simulink model "initializejoystick_model"  (Simulink 6.4)
settings: Solver=ode4  StartTime=0.0  StopTime=0.02*100  FixedStep=0.02  RelTol=1e-3
libraries: aerosimlib x1, RT x1
Description:
  | This model is be used with InitializeJoystick.m in order to obtain appropriate zero offsets and gains for the joystick interface.
settings Model: Creator=Christopher Lum  LastModifiedBy=root
settings DataIOCC: SignalLoggingName=sigsOut
settings DebuggingCC: SolverPrmCheckMsg=none  StrictBusMsg=None
settings HardwareCC: TargetUnknown=on

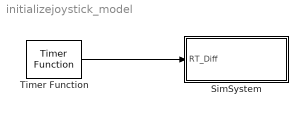
== system initializejoystick_model ==
  SimSystem : Subsystem
  Timer Function : RT/Timer Function  Priority=264547656  step=20  priority=HIGH  ThPriority=NORMAL
  wires:
  Timer Function/1 -> SimSystem/1(RT_Diff)

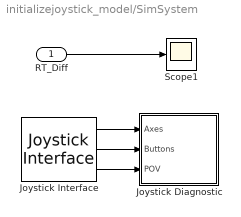
== system initializejoystick_model/SimSystem ==
  RT_Diff : Inport
  Joystick Diagnostic : Subsystem
  Joystick Interface : aerosimlib/Pilot Interface/Joystick Interface  SystemSampleTime=-1  joyid=1  tsamp=0.02
  Scope1 : Scope
      settings: YMin=0  YMax=4500
  wires:
  RT_Diff/1 -> Scope1/1
  Joystick Interface/1 -> Joystick Diagnostic/1(Axes)
  Joystick Interface/2 -> Joystick Diagnostic/2(Buttons)
  Joystick Interface/3 -> Joystick Diagnostic/3(POV)

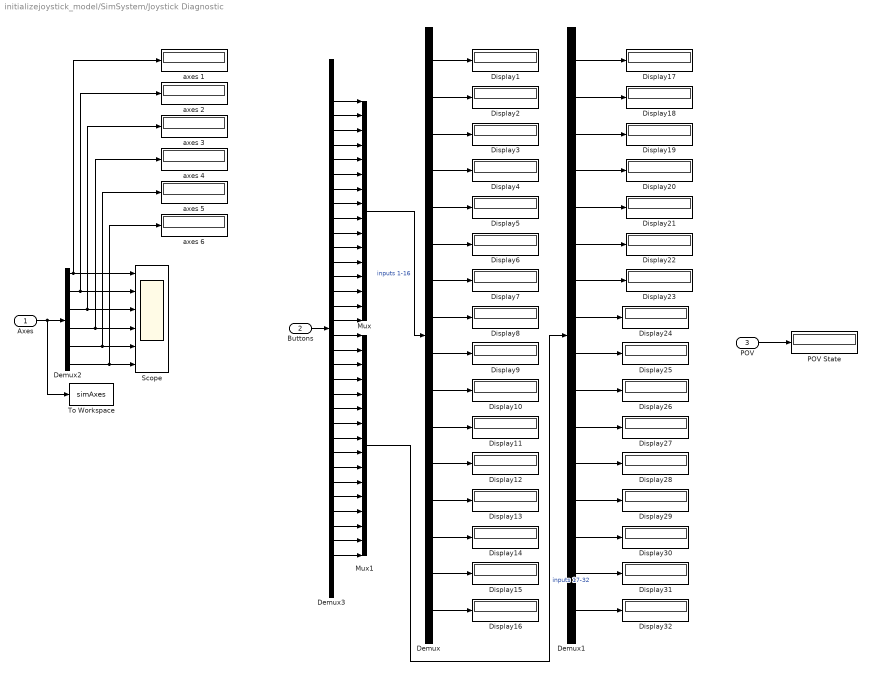
== system initializejoystick_model/SimSystem/Joystick Diagnostic ==
  Axes : Inport
  Buttons : Inport  Port=2
  POV : Inport  Port=3
  Demux : Demux  Outputs=16
  Demux1 : Demux  Outputs=16
  Demux2 : Demux  Outputs=6
  Demux3 : Demux  Outputs=32
  Display{1..32} (32 alike) : Display
  Mux : Mux  Inputs=16
  Mux1 : Mux  Inputs=16
  POV State : Display
  Scope : Scope  NumInputPorts=6
      settings: YMin=30885.5~30885.5~62258.3~-1~-1~-1  YMax=34136.6~34136.6~68811.8~1~1~1
  To Workspace : ToWorkspace  VariableName=simAxes  SampleTime=-1  SaveFormat=Structure With Time
  axes {1..6} (6 alike) : Display
  wires:
  Buttons/1 -> Demux3/1
  Demux3/1 -> Mux/1
  Demux3/2 -> Mux/2
  Demux3/3 -> Mux/3
  Demux3/4 -> Mux/4
  Demux3/5 -> Mux/5
  Demux3/6 -> Mux/6
  Demux3/7 -> Mux/7
  Demux3/8 -> Mux/8
  Demux3/9 -> Mux/9
  Demux3/10 -> Mux/10
  Demux3/11 -> Mux/11
  Demux3/12 -> Mux/12
  Demux3/13 -> Mux/13
  Demux3/14 -> Mux/14
  Demux3/15 -> Mux/15
  Demux3/16 -> Mux/16
  Mux/1 -> Demux/1  "inputs 1-16"
  Demux3/17 -> Mux1/1
  Demux3/18 -> Mux1/2
  Demux3/19 -> Mux1/3
  Demux3/20 -> Mux1/4
  Demux3/21 -> Mux1/5
  Demux3/22 -> Mux1/6
  Demux3/23 -> Mux1/7
  Demux3/24 -> Mux1/8
  Demux3/25 -> Mux1/9
  Demux3/26 -> Mux1/10
  Demux3/27 -> Mux1/11
  Demux3/28 -> Mux1/12
  Demux3/29 -> Mux1/13
  Demux3/30 -> Mux1/14
  Demux3/31 -> Mux1/15
  Demux3/32 -> Mux1/16
  Mux1/1 -> Demux1/1  "inputs 17-32"
  Demux/1 -> Display1/1
  Demux/2 -> Display2/1
  Demux/3 -> Display3/1
  Demux/4 -> Display4/1
  Demux/5 -> Display5/1
  Demux/6 -> Display6/1
  Demux/7 -> Display7/1
  Demux/8 -> Display8/1
  Demux/9 -> Display9/1
  Demux/10 -> Display10/1
  Demux/11 -> Display11/1
  Demux/12 -> Display12/1
  Demux/13 -> Display13/1
  Demux/14 -> Display14/1
  Demux/15 -> Display15/1
  Demux/16 -> Display16/1
  Demux1/1 -> Display17/1
  Demux1/2 -> Display18/1
  Demux1/3 -> Display19/1
  Demux1/4 -> Display20/1
  Demux1/5 -> Display21/1
  Demux1/6 -> Display22/1
  Demux1/7 -> Display23/1
  Demux1/8 -> Display24/1
  Demux1/9 -> Display25/1
  Demux1/10 -> Display26/1
  Demux1/11 -> Display27/1
  Demux1/12 -> Display28/1
  Demux1/13 -> Display29/1
  Demux1/14 -> Display30/1
  Demux1/15 -> Display31/1
  Demux1/16 -> Display32/1
  Axes/1 -> Demux2/1, To Workspace/1
  Demux2/1 -> Scope/1, axes 1/1
  Demux2/2 -> Scope/2, axes 2/1
  Demux2/3 -> Scope/3, axes 3/1
  Demux2/4 -> Scope/4, axes 4/1
  Demux2/5 -> Scope/5, axes 5/1
  Demux2/6 -> Scope/6, axes 6/1
  POV/1 -> POV State/1
